simulink library "EmptyInterpretationEngine"  (R2022b)
settings: Solver=VariableStepAuto  StartTime=0.0  StopTime=10.0  RelTol=1e-3
libraries: StateVar x2, FeaturePath x1, TSP x1
settings Model: MAModelExclusionFileProxy=C:\work\talariaDev\module\talaria_check_exclusions.xml  Creator=kl13806  LastModifiedBy=kl13806
settings SolverCC: AlgebraicLoopSolver=TrustRegion
settings DebuggingCC: UnconnectedInputMsg=warning  UnconnectedOutputMsg=warning  UnconnectedLineMsg=warning  SFMachineParentedDataDiag=warning  ArithmeticOperatorsInVariantConditions=warning
settings ModelReferenceCC: EnableRefExpFcnMdlSchedulingChecks=on
settings SFSimCC: SimUseLocalCustomCode=off  CustomCodeUndefinedFunction=UseInterfaceOnly
settings RTWCC: RTWUseLocalCustomCode=off  DLArmComputeVersion=19.05

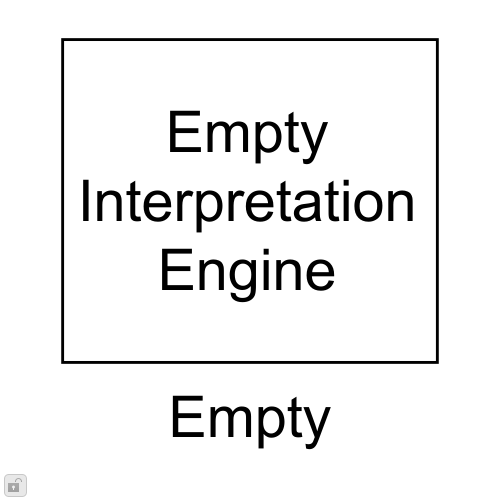
[thumbnail: Simulink's stored preview of the top-level diagram]
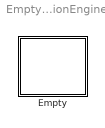
== system EmptyInterpretationEngine ==
  Empty : Subsystem  mask(Talaria Empty Interpretation Engine){}
      mask Display: disp(['Empty' newline 'Interpretation' newline 'Engine']);

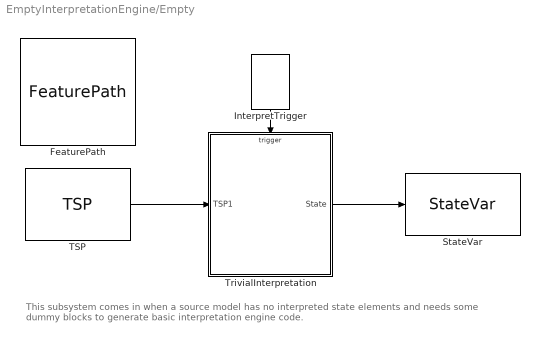
== system EmptyInterpretationEngine/Empty ==
  note: This subsystem comes in when a source model has
      | no interpreted state elements and needs some dummy
      | blocks to generate basic interpretation engine code.
  FeaturePath : FeaturePath/FeaturePath  FeatureName=DUMMY_  IsGroup=off  GroupNumber=-1  IsModule=off  TriggerInit=[75 -61 190 46]
      settings: SourceProductName=Bose Talaria
  InterpretTrigger : StateVar/InterpretTrigger  TriggerInit=[306 -45 344 10]
      settings: SourceProductName=Bose Talaria
  StateVar : StateVar/StateVar  TriggerInit=[460 74 575 136]  StateName=EMPTY
      settings: SourceProductName=Bose Talaria
  TSP : TSP/TSP  TriggerInit=[80 69 185 141]  TspName=EMPTY  IfDefMacro=[]  Role=Automatic
      settings: SourceProductName=Bose Talaria
  TrivialInterpretation : MATLAB Function  TreatAsAtomicUnit=on  mask(Talaria Trivial Interpretation){}
  wires:
  InterpretTrigger/1 -> TrivialInterpretation/Trigger
  TSP/1 -> TrivialInterpretation/1(TSP1)
  TrivialInterpretation/1(State) -> StateVar/1

== matlab function EmptyInterpretationEngine/Empty/TrivialInterpretation ==
  data: State output; TSP1 input
  events: trigger input FUNCTION_CALL_EVENT
function State  = fcn(TSP1)
%#codegen

% Use one or more input Targe State Probes (TSP) or Captured State
% Constants to calculate an output state value that feeds into a StateVar
% block. Unlike tune translation code, this state interpretation code does
% not support variable size inputs - TSPs each have a fixed size. As a
% result, the input signals are just normal signal values that do *not*
% have .Value and .Size fields. No need for a custom bus!

% ----- To register an error, use the following method (works like printf):
%   InterpretError( <format string>, <arguments ... )
%   ... this error will cause the build process to abort.

% A trivial pass-through interpretation looks like this:
State = TSP1;
